simulink model "rtwdemo_mdlreftop"  (Simulink 6.0)
settings: Solver=FixedStepDiscrete  SolverMode=SingleTasking  StartTime=0.0  StopTime=10.0  FixedStep=0.1  RelTol=1e-3
settings Model: Creator=The MathWorks Inc.  LastModifiedBy=batserve  ExtModeAutoUpdateStatusClock=off  ProdHWDeviceType=Specified
settings DataIOCC: LimitDataPoints=off  SaveFormat=StructureWithTime  SaveOutput=off  SaveTime=off  SignalLoggingName=logsOut
settings OptimizationCC: InlineParams=on  EnforceIntegerDowncast=off  StateBitsets=on  DataBitsets=on  UseTempVars=on
settings DebuggingCC: CheckExecutionContextPreStartOutputMsg=on  CheckExecutionContextRuntimeOutputMsg=on  SignalResolutionControl=UseLocalSettings  SolverPrmCheckMsg=none
settings HardwareCC: ProdHWDeviceType=Specified  TargetHWDeviceType=32-bit Generic
settings ModelReferenceCC: UpdateModelReferenceTargets=IfOutOfDate  CheckModelReferenceTargetMessage=none
settings RTWCC: TLCOptions=-p0 -aWarnNonSaturatedBlocks=0  GenerateReport=on  RTWVerbose=off  ProcessScript=grt_make_rtw_hook  LaunchReport=on
settings CodeAppCC: ForceParamTrailComments=on

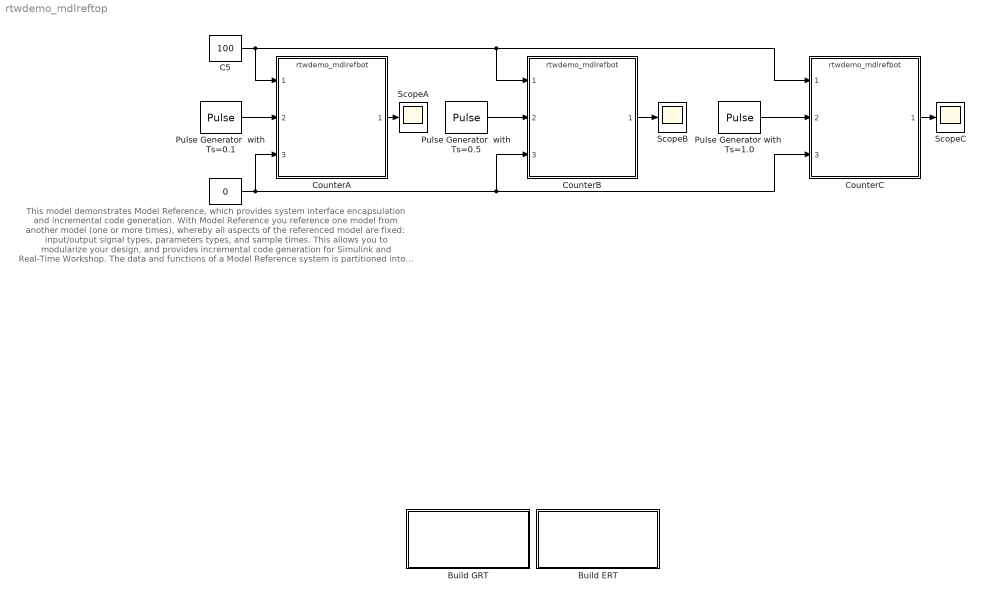
== system rtwdemo_mdlreftop ==
  note: This model demonstrates Model Reference, which provides system interface encapsulation and incremental code generation.
      | With Model Reference you reference one model from another model (one or more times), whereby all aspects of the referenced
      | model are fixed: input/output signal types, parameters types, and sample times.  This allows you to modularize your
      | design, and provides incremental code generation for Simulink and Real-Time Workshop.
      |
      | The data and functions of a Model Reference system is partitioned into its own set of files, independent of its parent
      | model.
      |
      | In this example, the model 'rtwdemo_mdlrefbot.mdl' is referenced three times.  For simulation and code generation, the
      | model is incrementally generated.  That is, rtwdemo_mdlrefbot.mdl will build the first time, but not on subsequent
      | builds (until rtwdemo_mdlrefbot.mdl is changed.)
      |
      | Since Model Reference shares and manages code for models, each RTW target must be built into its own directory.  The
      | blue buttons below generate the code into ./rtwdemo_grt and ./rtwdemo_ert for RTW and RTW-EC, respectively.
      |
      | For more demonstrations of Model Reference capabilities, particularly for specifying parameter arguments and signal
      | bus interfaces, type mdlrefdemos.
  Build ERT : Subsystem  AncestorBlock=rtwdemowidgets/Build ERT  PropExecContextAcrossSSBoundary=on  mask{attrib_overrides={'CustomSymbolStr'}}
      mask prompts: attrib_overrides "List of attributes to preserve (cell of strings):"
      mask help: Enter the attributes of the configuration set that you want preserved. Otherwise, the default configuration script will override your current settings.
      settings: OpenFcn=|
      | try
      |   if ~exist('rtwdemo_ert', 'dir')
      |     mkdir('rtwdemo_ert')
      |   end
      |   cd('rtwdemo_ert');
      |   overrides=get_param(gcb,'attrib_overrides');
      |   model='rtwdemo_mdlrefbot';
      |   load_system(model);
      |   rtwconfiguredemo(model,'noop',false,overrides);
      |   cs=getActiveConfigSet(model);
      |   set_param(cs,'CustomSymbolStr','$R$N$M');
      |   set_param(model,'dirty','off');
      |   model='rtwdemo_mdlreftop';
      |   rtwconfiguredemo(model,'noop',false,overrides);
      |   cs=getActiveConfigSet(model);
      |   set_param(cs,'CustomSymbolStr','$R$N$M');
      |   set_param(model,'dirty','off');
      |   rtwbuilddemomodel(model);
      |   cd('..')
      |   close_system('rtwdemo_mdlrefbot');
      | catch
      |   error(lasterr);
      | end
      mask Display:
      | disp(['Generate Code Using\n',...
      | 	  'Real-Time Workshop\n',...
      | 	  'Embedded Coder\n'...
      | 	  '(double-click)'])
  Build GRT : Subsystem  AncestorBlock=rtwdemowidgets/Build GRT  PropExecContextAcrossSSBoundary=on  mask{attrib_overrides={}}
      mask prompts: attrib_overrides "List of attributes to preserve (cell of strings):"
      mask help: Enter the attributes of the configuration set that you want preserved. Otherwise, the default configuration script will override your current settings.
      settings: OpenFcn=|
      | try
      |   if ~exist('rtwdemo_grt','dir')
      |     mkdir('rtwdemo_grt');
      |   end
      |   chdir('rtwdemo_grt')
      |   overrides=get_param(gcb,'attrib_overrides');
      |   model='rtwdemo_mdlrefbot';
      |   load_system(model);
      |   rtwconfiguredemo(model,'noop',true,overrides);
      |   model='rtwdemo_mdlreftop';
      |   rtwconfiguredemo(model,'noop',true,overrides);
      |   rtwbuilddemomodel(model);
      |   cd('..');
      | catch
      |   error(lasterr);
      | end
      mask Display:
      | disp(['Generate Code Using\n',...
      | 	  'Real-Time Workshop\n',...
      | 	  '(double-click)'])
  C1 : Constant  Value=0
  C5 : Constant  Value=100
  CounterA : ModelReference  ModelName=rtwdemo_mdlrefbot  ModelReferenceVersion=1.67  CopyOfModelName=rtwdemo_mdlrefbot
  CounterB : ModelReference  ModelName=rtwdemo_mdlrefbot  ModelReferenceVersion=1.67  CopyOfModelName=rtwdemo_mdlrefbot
  CounterC : ModelReference  ModelName=rtwdemo_mdlrefbot  ModelReferenceVersion=1.67  CopyOfModelName=rtwdemo_mdlrefbot
  Pulse Generator  with Ts=0.1 : DiscretePulseGenerator  SampleTime=0.1  VectorParams1D=off
  Pulse Generator  with Ts=0.5 : DiscretePulseGenerator  SampleTime=0.5
  Pulse Generator with  Ts=1.0 : DiscretePulseGenerator  SampleTime=1.0
  ScopeA : Scope
      settings: TimeRange=10  YMin=0  YMax=100
  ScopeB : Scope
      settings: TimeRange=10  YMin=0  YMax=25
  ScopeC : Scope
      settings: TimeRange=10  YMin=0  YMax=15  SaveName=ScopeData2
  wires:
  CounterB/1 -> ScopeB/1
  CounterA/1 -> ScopeA/1
  CounterC/1 -> ScopeC/1
  Pulse Generator  with Ts=0.1/1 -> CounterA/2
  Pulse Generator  with Ts=0.5/1 -> CounterB/2
  Pulse Generator with  Ts=1.0/1 -> CounterC/2
  C1/1 -> CounterC/3, CounterB/3, CounterA/3
  C5/1 -> CounterA/1, CounterB/1, CounterC/1

== system rtwdemo_mdlreftop/Build ERT ==

== system rtwdemo_mdlreftop/Build GRT ==
